simulink model "BoostConverterDoubleLoopControl"  (R2024b)
settings: Solver=ode45  StartTime=0.0  StopTime=0.1  MaxStep=1e-4  RelTol=1e-3
undefined symbols (not defined in the file or in its folder): Ion, Lithium
libraries: spsSeriesRLCBranchLib x5, spsCurrentMeasurementLib x3, spsVoltageMeasurementLib x2, spsBreakerLib x2, spsIGBTDiodeLib x2, spsBatteryLib x1, spsMeanLib x1, spsPWMGeneratorDCDCLib x1, sps_lib x1
settings Model: Creator=user  LastModifiedBy=User
settings SolverCC: AlgebraicLoopSolver=TrustRegion
settings DataIOCC: ReturnWorkspaceOutputs=off
settings DebuggingCC: UnconnectedInputMsg=warning  UnconnectedOutputMsg=warning  UnconnectedLineMsg=warning  ArithmeticOperatorsInVariantConditions=warning
settings ModelReferenceCC: EnableRefExpFcnMdlSchedulingChecks=on
settings SFSimCC: SimUseLocalCustomCode=off  CustomCodeUndefinedFunction=UseInterfaceOnly
settings RTWCC: RTWUseLocalCustomCode=off  GPUComputeCapability=3.5

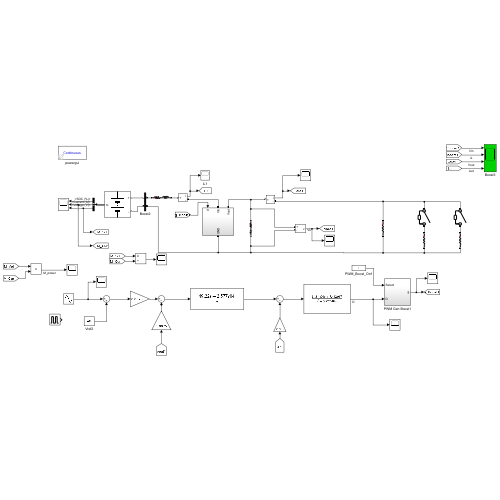
[thumbnail: Simulink's stored preview of the top-level diagram]
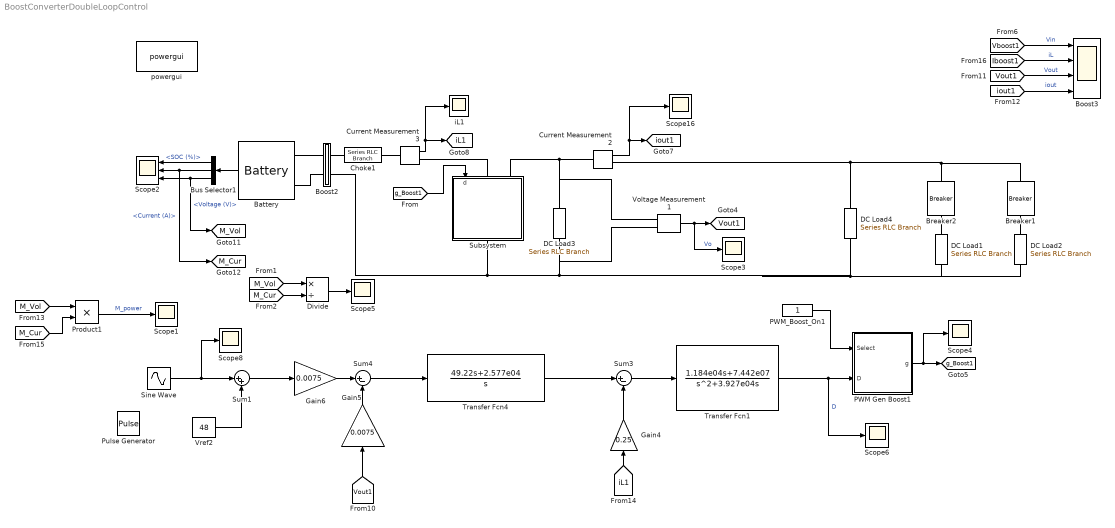
== system BoostConverterDoubleLoopControl ==
  Battery : spsBatteryLib/Battery  BatType=Lithium-Ion  NomV=25  NomQ=50  SOC=90  Batt_Tr=30  PresetModel=on  MaxQ=50  MinV=18.75  FullV=29.0997  Dis_rate=21.7391  R=0.005  Normal_OP=45.2174  expZone="[27.0096      2.45652]"
      settings: LibrarySourceBlock=electricdrivelib/Extra Sources/Battery
  Boost2 : Subsystem
  Boost3 : Scope  NumInputPorts=4
  Breaker1 : spsBreakerLib/Breaker  InitialState=0  SwitchingTimes=[0.2]  External=off  BreakerResistance=0.0001  SnubberResistance=1e6  SnubberCapacitance=inf  Measurements=None  MoreParameters=on  NoBreakLoop=off
  Breaker2 : spsBreakerLib/Breaker  InitialState=0  SwitchingTimes=[0.1]  External=off  BreakerResistance=0.0001  SnubberResistance=1e6  SnubberCapacitance=inf  Measurements=None  MoreParameters=on  NoBreakLoop=off
  Bus Selector1 : BusSelector  OutputSignals=SOC (%),Current (A),Voltage (V)
  Choke1 : spsSeriesRLCBranchLib/Series RLC Branch  LConnTagsString=__new0  RConnTagsString=__new0  BranchType=RL  Resistance=10e-3  Inductance=240e-6  SetiL0=off  InitialCurrent=0  Capacitance=1e-6  Setx0=off  InitialVoltage=0  Measurements=None
  Current Measurement2 : spsCurrentMeasurementLib/Current Measurement  PhasorSimulation=off  OutputType=Complex  PSBequivalent=0
  Current Measurement3 : spsCurrentMeasurementLib/Current Measurement  PhasorSimulation=off  OutputType=Complex  PSBequivalent=0
  DC Load1 : spsSeriesRLCBranchLib/Series RLC Branch  LConnTagsString=__new0  RConnTagsString=__new0  BranchType=R  Resistance=100  Inductance=10e-5  SetiL0=off  InitialCurrent=0  Capacitance=1e-6  Setx0=off  InitialVoltage=0  Measurements=None
  DC Load2 : spsSeriesRLCBranchLib/Series RLC Branch  LConnTagsString=__new0  RConnTagsString=__new0  BranchType=R  Resistance=100  Inductance=10e-5  SetiL0=off  InitialCurrent=0  Capacitance=1e-6  Setx0=off  InitialVoltage=0  Measurements=None
  DC Load3 : spsSeriesRLCBranchLib/Series RLC Branch  LConnTagsString=__new0  RConnTagsString=__new0  BranchType=RC  Resistance=0.01  Inductance=1e-3  SetiL0=off  InitialCurrent=0  Capacitance=100e-6  Setx0=on  InitialVoltage=48  Measurements=None
  DC Load4 : spsSeriesRLCBranchLib/Series RLC Branch  LConnTagsString=__new0  RConnTagsString=__new0  BranchType=R  Resistance=100  Inductance=10e-5  SetiL0=off  InitialCurrent=0  Capacitance=1e-6  Setx0=off  InitialVoltage=0  Measurements=None
  Divide : Product  Inputs=*/
  Gain4 : Gain  Gain=0.25
  Gain5 : Gain  Gain=0.0075
  Gain6 : Gain  Gain=0.0075
  PWM Gen Boost1 : Subsystem
  PWM_Boost_On1 : Constant
  Product1 : Product
  Pulse Generator : DiscretePulseGenerator  PulseType=Time based  Amplitude=3  Period=1/100  PulseWidth=50
  Scope{1,3..6,8,16} (7 alike) : Scope
  Scope2 : Scope  NumInputPorts=3
  Sine Wave : Sin  Amplitude=2  Frequency=2*pi*100  SampleTime=0
  Subsystem : Subsystem
  Sum1 : Sum  Inputs=|++
  Sum3 : Sum  Inputs=|+-
  Sum4 : Sum  Inputs=|+-
  Transfer Fcn1 : TransferFcn  Numerator=[1.184e04 7.442e07]  Denominator=[1 3.927e04 0]
  Transfer Fcn4 : TransferFcn  Numerator=[49.22 2.577e04]  Denominator=[1 0]
  Voltage Measurement1 : spsVoltageMeasurementLib/Voltage Measurement  PhasorSimulation=off  OutputType=Complex  PSBequivalent=0
  Vref2 : Constant  Value=48
  iL1 : Scope
  powergui : sps_lib/powergui  Priority=1  SimulationMode=Continuous  SampleTime=5e-7  frequency=60  Iterations=50  frequencyindice=0  Pbase=100e6  ErrMax=1e-4  UnitsV=kV  UnitsW=MW  buscounter=0  FunctionMessages=off  echomessages=off  EnableUseOfTLC=off  CurrentSourceSwitches=off  DisableSnubberDevices=off  DisableRonSwitches=off  DisableVfSwitches=off  DisplayEquations=off  AutomaticDiscreteSolvers=off  SolverType=Tustin/Backward Euler (TBE)  Interpol=off  ExternalGateDelay=off  methode=off  Ts=100  x0status=blocks  SPID=on  SwTol=0  HookPort=off  NonlinearTolerance=1e-4  nMaxIteration=100  ContinueOnMaxIteration=off  RestoreLinks=warning  ResistiveCurrentMeasurement=off  Frange=[0:2:500]  Ylog=off  Xlog=on  ShowGrid=off  save=off  variable=ZData  structure=0  ZoomFFT=off  StartTime=0.0  cycles=1  DisplayStyle=1  fundamental=60  FreqAxis=off  MaxFrequency=1000  frequencyindicesteady=1  RmsSteady=1  display=off
  tag scope: M_Cur=global, M_Vol=global, Vout1=global, g_Boost1=global, iL1=global, iout1=global
  wires:
  Transfer Fcn1/1 -> Scope6/1, PWM Gen Boost1/2(D)  "D"
  Bus Selector1/1 -> Scope2/1  "<SOC (%)>"
  Gain4/1 -> Sum3/2
  [Vout1] -> Gain5/1
  [Vboost1] -> Boost3/1  "Vin"
  Product1/1 -> Scope1/1  "M_power"
  [M_Cur] -> Product1/2
  Current Measurement3/1 -> iL1/1, [iL1]
  Bus Selector1/3 -> [M_Vol], Scope2/3  "<Voltage (V)>"
  [Iboost1] -> Boost3/2  "iL"
  [iout1] -> Boost3/4  "iout"
  Sum3/1 -> Transfer Fcn1/1
  Battery/1 -> Bus Selector1/1
  PWM_Boost_On1/1 -> PWM Gen Boost1/1(Select)
  [M_Vol] -> Product1/1
  Sum4/1 -> Transfer Fcn4/1
  [Vout1] -> Boost3/3  "Vout"
  Gain5/1 -> Sum4/2
  Voltage Measurement1/1 -> Scope3/1, [Vout1]  "Vo"
  Bus Selector1/2 -> [M_Cur], Scope2/2  "<Current (A)>"
  Current Measurement2/1 -> [iout1], Scope16/1
  PWM Gen Boost1/1(g) -> [g_Boost1], Scope4/1
  [g_Boost1] -> Subsystem/1(d)
  Gain6/1 -> Sum4/1
  [iL1] -> Gain4/1
  Vref2/1 -> Sum1/2
  [M_Vol] -> Divide/1
  [M_Cur] -> Divide/2
  Divide/1 -> Scope5/1
  Transfer Fcn4/1 -> Sum3/1
  Sum1/1 -> Gain6/1
  Sine Wave/1 -> Scope8/1, Sum1/1
  connections:
  Boost2/RConn2 -- DC Load2/RConn1 -- DC Load1/RConn1 -- DC Load4/RConn1 -- Voltage Measurement1/LConn2 -- DC Load3/RConn1 -- Subsystem/RConn1
  Boost2/RConn1 -- Choke1/LConn1
  Current Measurement3/LConn1 -- Choke1/RConn1
  Breaker2/LConn1 -- Breaker1/LConn1 -- DC Load4/LConn1 -- Current Measurement2/RConn1
  Breaker1/RConn1 -- DC Load2/LConn1
  Current Measurement3/RConn1 -- Subsystem/LConn1
  Breaker2/RConn1 -- DC Load1/LConn1
  Battery/LConn1 -- Boost2/LConn1
  Current Measurement2/LConn1 -- Voltage Measurement1/LConn1 -- DC Load3/LConn1 -- Subsystem/LConn2
  Battery/LConn2 -- Boost2/LConn2

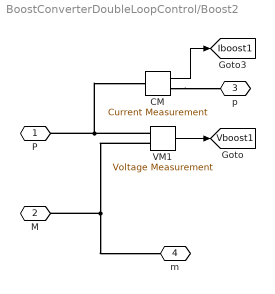
== system BoostConverterDoubleLoopControl/Boost2 ==
  CM : spsCurrentMeasurementLib/Current Measurement  PhasorSimulation=off  OutputType=Complex  PSBequivalent=0
  VM1 : spsVoltageMeasurementLib/Voltage Measurement  PhasorSimulation=off  OutputType=Complex  PSBequivalent=0
  P : PMIOPort  Side=Left
  M : PMIOPort  Port=2  Side=Left
  p : PMIOPort  Port=3  Side=Right
  m : PMIOPort  Port=4  Side=Right
  tag scope: Iboost1=global, Vboost1=global
  wires:
  VM1/1 -> [Vboost1]
  CM/1 -> [Iboost1]
  connections:
  VM1/LConn1 -- CM/LConn1 -- P/RConn1
  VM1/LConn2 -- m/RConn1 -- M/RConn1
  CM/RConn1 -- p/RConn1

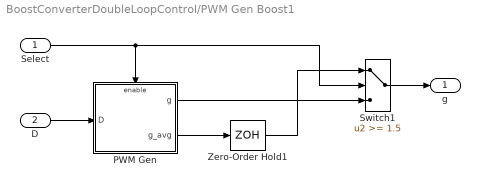
== system BoostConverterDoubleLoopControl/PWM Gen Boost1 ==
  Select : Inport
  D : Inport  Port=2
  PWM Gen : Subsystem
  Switch1 : Switch  Threshold=1.5  SaturateOnIntegerOverflow=off  InputSameDT=off
  Zero-Order Hold1 : ZeroOrderHold  SampleTime=5e-7
  g : Outport  VectorParamsAs1DForOutWhenUnconnected=off
  wires:
  D/1 -> PWM Gen/1(D)
  Select/1 -> Switch1/2, PWM Gen/Enable
  Switch1/1 -> g/1
  PWM Gen/1(g) -> Switch1/3
  PWM Gen/2(g_avg) -> Zero-Order Hold1/1
  Zero-Order Hold1/1 -> Switch1/1

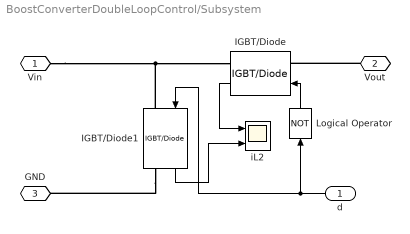
== system BoostConverterDoubleLoopControl/Subsystem ==
  d : Inport
  IGBT/Diode : spsIGBTDiodeLib/IGBT//Diode  Ron=1e-3  Rs=1e5  Cs=inf  Measurements=on
  IGBT/Diode1 : spsIGBTDiodeLib/IGBT//Diode  Ron=1e-3  Rs=1e5  Cs=inf  Measurements=on
  Logical Operator : Logic  Operator=NOT  AllPortsSameDT=off  OutDataTypeStr=float('double')
  iL2 : Scope  NumInputPorts=2
  Vin : PMIOPort  Side=Left
  Vout : PMIOPort  Port=2  Side=Left
  GND : PMIOPort  Port=3  Side=Right
  wires:
  IGBT/Diode1/1 -> iL2/2
  Logical Operator/1 -> IGBT/Diode/1
  d/1 -> IGBT/Diode1/1, Logical Operator/1
  IGBT/Diode/1 -> iL2/1
  connections:
  IGBT/Diode1/RConn1 -- GND/RConn1
  Vin/RConn1 -- IGBT/Diode1/LConn1 -- IGBT/Diode/RConn1
  Vout/RConn1 -- IGBT/Diode/LConn1

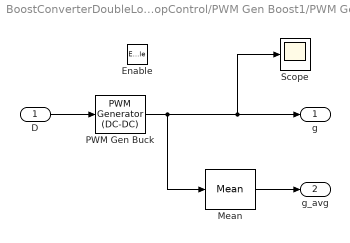
== system BoostConverterDoubleLoopControl/PWM Gen Boost1/PWM Gen ==
  D : Inport
  Enable : EnablePort
  Mean : spsMeanLib/Mean  Freq=1/5e-7  Vinit=0  Ts=5e-7
  "PWM Gen Buck " : spsPWMGeneratorDCDCLib/PWM Generator (DC-DC)  Fsw=25e03  Ts=5e-7
  Scope : Scope
  g : Outport  VectorParamsAs1DForOutWhenUnconnected=off
  g_avg : Outport  Port=2  VectorParamsAs1DForOutWhenUnconnected=off
  wires:
  "PWM Gen Buck "/1 -> Scope/1, g/1, Mean/1
  D/1 -> "PWM Gen Buck "/1
  Mean/1 -> g_avg/1
